simulink subsystem "ScannerBank"  (R2025b)
settings: Solver=VariableStepAuto  StartTime=0.0  StopTime=10.0  RelTol=1e-3
values from neighbouring files (symbols this model uses):
  m = min(v)    [run_loader_scanner_model_multi_stress_v1_2_final_verified.m]    (also in run_slide_model_daily_scenarios_v2.m; run_slide_model_daily_scenarios_v2_scannerbank_v2.m)
  ScannerEnabled = logical(S(testIdx).enabled(:).')    [run_loader_scanner_model_multi_stress_v1_2_final_verified.m]    (also in run_slide_model_daily_scenarios_v2_scannerbank_v2.m = false(1,n_physical_scanners))
  Total_Scanner_Rack_Slots_Available = nActiveScanners * Scanner_RackQueueSize    [run_loader_scanner_model_multi_stress_v1_2_final_verified.m]    (also in run_slide_model_daily_scenarios_v2.m = n_active_scanners * Scanner_RackQueueSize; run_slide_model_daily_scenarios_v2_scannerbank_v2.m = nnz(ScannerEnabled) * Scanner_RackQueueSize)
settings Model: Creator=bayes  LastModifiedBy=bayes

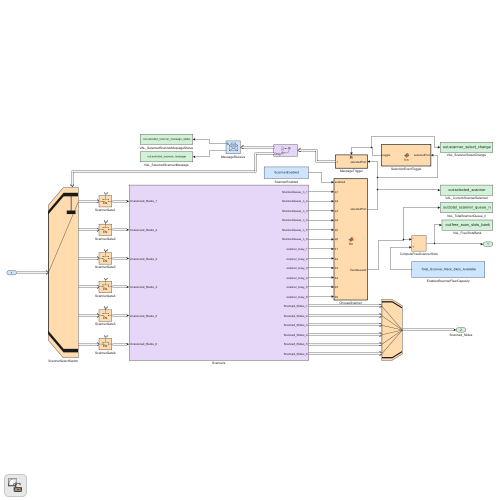
[thumbnail: Simulink's stored preview of the top-level diagram]
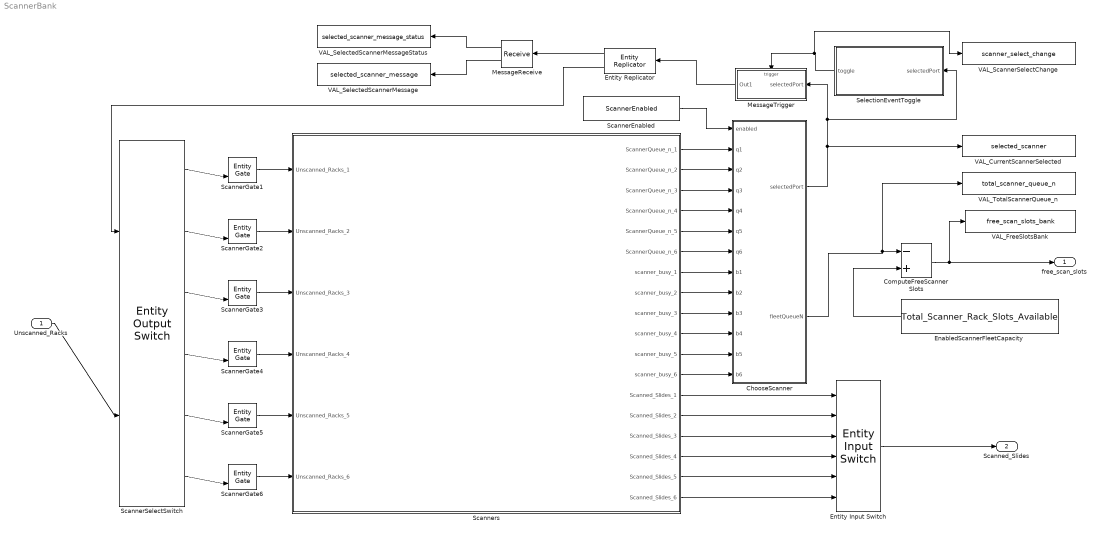
== system ScannerBank ==
  Unscanned_Racks : Inport
  ChooseScanner : MATLAB Function  TreatAsAtomicUnit=on
  ComputeFreeScannerSlots : Sum  Inputs=-+
  EnabledScannerFleetCapacity : Constant  Value=Total_Scanner_Rack_Slots_Available  OutMin=0
  Entity Input Switch : EntityInputSwitch  InputPortMessageModes=m,m,m,m,m,m  OutputPortMessageModes=m  NumberInputPorts=6
      settings: InputPortMap=u1,u2,u3,u4,u5,u6
  Entity Replicator : EntityReplicator  InputPortMessageModes=m  OutputPortMessageModes=m,m  HoldOriginalEntityUntilAllReplicasDepart=on
  MessageReceive : Receive  InputPortMessageModes=m  ShowQueueStatus=on  InitialValue=0  ValueSourceWhenQueueIsEmpty=Use initial value
      settings: OutputPortMap=o0,o1
  MessageTrigger : Subsystem  TreatAsAtomicUnit=on
  ScannerEnabled : Constant  Value=ScannerEnabled
  ScannerGate{1..6} (6 alike) : EntityGate  InputPortMessageModes=m,m  OutputPortMessageModes=m  OpenGateAtSimulationStart=on
  ScannerSelectSwitch : EntityOutputSwitch  InputPortMessageModes=m,m  OutputPortMessageModes=m,m,m,m,m,m  NumberOutputPorts=6  SwitchingCriterion=From control port  SwitchAttributeName=Attribute1
      settings: InputPortMap=u0,u1  OutputPortMap=o0,o1,o2,o3,o4,o5
  Scanners : Subsystem
  SelectionEventToggle : MATLAB Function  TreatAsAtomicUnit=on
  VAL_CurrentScannerSelected : ToWorkspace  VariableName=selected_scanner  SaveFormat=Timeseries  SampleTime=-1
  VAL_FreeSlotsBank : ToWorkspace  VariableName=free_scan_slots_bank  SaveFormat=Timeseries  SampleTime=-1
  VAL_ScannerSelectChange : ToWorkspace  VariableName=scanner_select_change  SaveFormat=Timeseries  SampleTime=-1
  VAL_SelectedScannerMessage : ToWorkspace  VariableName=selected_scanner_message  SaveFormat=Timeseries  SampleTime=-1
  VAL_SelectedScannerMessageStatus : ToWorkspace  VariableName=selected_scanner_message_status  SaveFormat=Timeseries  SampleTime=-1
  VAL_TotalScannerQueue_n : ToWorkspace  VariableName=total_scanner_queue_n  SaveFormat=Timeseries  SampleTime=-1
  free_scan_slots : Outport
  Scanned_Slides : Outport  Port=2
  wires:
  Scanners/2(ScannerQueue_n_2) -> ChooseScanner/3(q2)
  Scanners/9(scanner_busy_3) -> ChooseScanner/10(b3)
  Scanners/1(ScannerQueue_n_1) -> ChooseScanner/2(q1)
  Entity Replicator/2 -> ScannerSelectSwitch/1
  Scanners/16(Scanned_Slides_4) -> Entity Input Switch/4
  ScannerGate4/1 -> Scanners/4(Unscanned_Racks_4)
  Scanners/6(ScannerQueue_n_6) -> ChooseScanner/7(q6)
  MessageTrigger/1(Out1) -> Entity Replicator/1
  ScannerSelectSwitch/4 -> ScannerGate4/2
  ScannerSelectSwitch/6 -> ScannerGate6/2
  ScannerGate2/1 -> Scanners/2(Unscanned_Racks_2)
  ScannerGate1/1 -> Scanners/1(Unscanned_Racks_1)
  ChooseScanner/1(selectedPort) -> SelectionEventToggle/1(selectedPort), MessageTrigger/1(selectedPort), VAL_CurrentScannerSelected/1
  ScannerGate5/1 -> Scanners/5(Unscanned_Racks_5)
  Scanners/13(Scanned_Slides_1) -> Entity Input Switch/1
  EnabledScannerFleetCapacity/1 -> ComputeFreeScannerSlots/2
  ScannerSelectSwitch/5 -> ScannerGate5/2
  ScannerSelectSwitch/2 -> ScannerGate2/2
  Scanners/18(Scanned_Slides_6) -> Entity Input Switch/6
  Entity Input Switch/1 -> Scanned_Slides/1
  MessageReceive/1 -> VAL_SelectedScannerMessageStatus/1
  Entity Replicator/1 -> MessageReceive/1
  ScannerSelectSwitch/3 -> ScannerGate3/2
  Unscanned_Racks/1 -> ScannerSelectSwitch/2
  Scanners/5(ScannerQueue_n_5) -> ChooseScanner/6(q5)
  Scanners/11(scanner_busy_5) -> ChooseScanner/12(b5)
  ComputeFreeScannerSlots/1 -> free_scan_slots/1, VAL_FreeSlotsBank/1
  Scanners/14(Scanned_Slides_2) -> Entity Input Switch/2
  Scanners/8(scanner_busy_2) -> ChooseScanner/9(b2)
  ScannerSelectSwitch/1 -> ScannerGate1/2
  Scanners/12(scanner_busy_6) -> ChooseScanner/13(b6)
  MessageReceive/2 -> VAL_SelectedScannerMessage/1
  Scanners/4(ScannerQueue_n_4) -> ChooseScanner/5(q4)
  ScannerGate3/1 -> Scanners/3(Unscanned_Racks_3)
  Scanners/15(Scanned_Slides_3) -> Entity Input Switch/3
  Scanners/7(scanner_busy_1) -> ChooseScanner/8(b1)
  ChooseScanner/2(fleetQueueN) -> ComputeFreeScannerSlots/1, VAL_TotalScannerQueue_n/1
  Scanners/10(scanner_busy_4) -> ChooseScanner/11(b4)
  Scanners/17(Scanned_Slides_5) -> Entity Input Switch/5
  ScannerGate6/1 -> Scanners/6(Unscanned_Racks_6)
  ScannerEnabled/1 -> ChooseScanner/1(enabled)
  SelectionEventToggle/1(toggle) -> MessageTrigger/Trigger, VAL_ScannerSelectChange/1
  Scanners/3(ScannerQueue_n_3) -> ChooseScanner/4(q3)

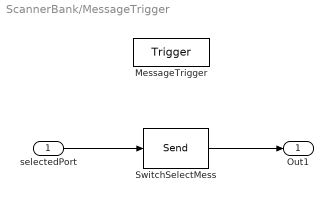
== system ScannerBank/MessageTrigger ==
  selectedPort : Inport
  MessageTrigger : TriggerPort  TriggerType=either  VariantControl=(inherit)
  SwitchSelectMess : Send  OutputPortMessageModes=m
  Out1 : Outport
  wires:
  SwitchSelectMess/1 -> Out1/1
  selectedPort/1 -> SwitchSelectMess/1

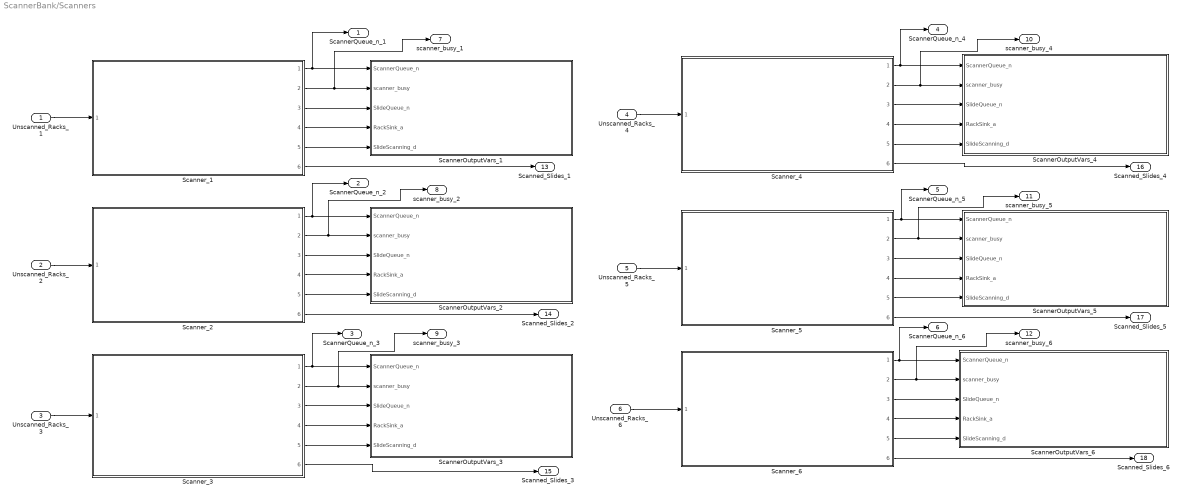
== system ScannerBank/Scanners ==
  Unscanned_Racks_1 : Inport
  Unscanned_Racks_2 : Inport  Port=2
  Unscanned_Racks_3 : Inport  Port=3
  Unscanned_Racks_4 : Inport  Port=4
  Unscanned_Racks_5 : Inport  Port=5
  Unscanned_Racks_6 : Inport  Port=6
  ScannerOutputVars_1 : Subsystem
  ScannerOutputVars_2 : Subsystem
  ScannerOutputVars_3 : Subsystem
  ScannerOutputVars_4 : Subsystem
  ScannerOutputVars_5 : Subsystem
  ScannerOutputVars_6 : Subsystem
  Scanner_{1..6} (6 alike) : Subsystem  ReferencedSubsystem=GenericScanner
  ScannerQueue_n_1 : Outport
  ScannerQueue_n_2 : Outport  Port=2
  ScannerQueue_n_3 : Outport  Port=3
  ScannerQueue_n_4 : Outport  Port=4
  ScannerQueue_n_5 : Outport  Port=5
  ScannerQueue_n_6 : Outport  Port=6
  scanner_busy_1 : Outport  Port=7
  scanner_busy_2 : Outport  Port=8
  scanner_busy_3 : Outport  Port=9
  scanner_busy_4 : Outport  Port=10
  scanner_busy_5 : Outport  Port=11
  scanner_busy_6 : Outport  Port=12
  Scanned_Slides_1 : Outport  Port=13
  Scanned_Slides_2 : Outport  Port=14
  Scanned_Slides_3 : Outport  Port=15
  Scanned_Slides_4 : Outport  Port=16
  Scanned_Slides_5 : Outport  Port=17
  Scanned_Slides_6 : Outport  Port=18
  wires:
  Scanner_2/6 -> Scanned_Slides_2/1
  Unscanned_Racks_4/1 -> Scanner_4/1
  Unscanned_Racks_1/1 -> Scanner_1/1
  Unscanned_Racks_6/1 -> Scanner_6/1
  Scanner_5/3 -> ScannerOutputVars_5/3(SlideQueue_n)
  Unscanned_Racks_3/1 -> Scanner_3/1
  Scanner_5/4 -> ScannerOutputVars_5/4(RackSink_a)
  Scanner_5/2 -> scanner_busy_5/1, ScannerOutputVars_5/2(scanner_busy)
  Scanner_2/4 -> ScannerOutputVars_2/4(RackSink_a)
  Scanner_1/6 -> Scanned_Slides_1/1
  Scanner_3/5 -> ScannerOutputVars_3/5(SlideScanning_d)
  Scanner_6/6 -> Scanned_Slides_6/1
  Scanner_3/4 -> ScannerOutputVars_3/4(RackSink_a)
  Scanner_1/3 -> ScannerOutputVars_1/3(SlideQueue_n)
  Scanner_6/4 -> ScannerOutputVars_6/4(RackSink_a)
  Scanner_2/2 -> scanner_busy_2/1, ScannerOutputVars_2/2(scanner_busy)
  Scanner_6/1 -> ScannerOutputVars_6/1(ScannerQueue_n), ScannerQueue_n_6/1
  Scanner_6/3 -> ScannerOutputVars_6/3(SlideQueue_n)
  Scanner_2/1 -> ScannerOutputVars_2/1(ScannerQueue_n), ScannerQueue_n_2/1
  Scanner_5/5 -> ScannerOutputVars_5/5(SlideScanning_d)
  Scanner_4/3 -> ScannerOutputVars_4/3(SlideQueue_n)
  Scanner_1/1 -> ScannerQueue_n_1/1, ScannerOutputVars_1/1(ScannerQueue_n)
  Scanner_6/5 -> ScannerOutputVars_6/5(SlideScanning_d)
  Scanner_4/1 -> ScannerOutputVars_4/1(ScannerQueue_n), ScannerQueue_n_4/1
  Scanner_4/5 -> ScannerOutputVars_4/5(SlideScanning_d)
  Scanner_3/2 -> ScannerOutputVars_3/2(scanner_busy), scanner_busy_3/1
  Unscanned_Racks_5/1 -> Scanner_5/1
  Scanner_6/2 -> scanner_busy_6/1, ScannerOutputVars_6/2(scanner_busy)
  Scanner_4/4 -> ScannerOutputVars_4/4(RackSink_a)
  Scanner_5/6 -> Scanned_Slides_5/1
  Scanner_3/6 -> Scanned_Slides_3/1
  Scanner_4/6 -> Scanned_Slides_4/1
  Scanner_1/2 -> ScannerOutputVars_1/2(scanner_busy), scanner_busy_1/1
  Scanner_5/1 -> ScannerOutputVars_5/1(ScannerQueue_n), ScannerQueue_n_5/1
  Scanner_4/2 -> scanner_busy_4/1, ScannerOutputVars_4/2(scanner_busy)
  Unscanned_Racks_2/1 -> Scanner_2/1
  Scanner_2/5 -> ScannerOutputVars_2/5(SlideScanning_d)
  Scanner_2/3 -> ScannerOutputVars_2/3(SlideQueue_n)
  Scanner_3/3 -> ScannerOutputVars_3/3(SlideQueue_n)
  Scanner_3/1 -> ScannerOutputVars_3/1(ScannerQueue_n), ScannerQueue_n_3/1
  Scanner_1/5 -> ScannerOutputVars_1/5(SlideScanning_d)
  Scanner_1/4 -> ScannerOutputVars_1/4(RackSink_a)

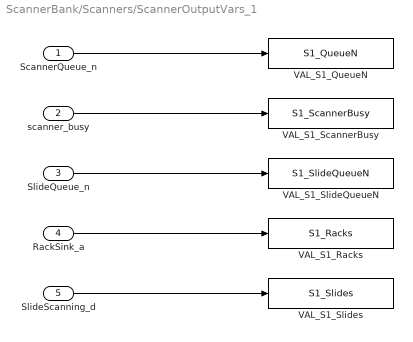
== system ScannerBank/Scanners/ScannerOutputVars_1 ==
  ScannerQueue_n : Inport
  scanner_busy : Inport  Port=2
  SlideQueue_n : Inport  Port=3
  RackSink_a : Inport  Port=4
  SlideScanning_d : Inport  Port=5
  VAL_S1_QueueN : ToWorkspace  VariableName=S1_QueueN  SaveFormat=Timeseries  SampleTime=-1
  VAL_S1_Racks : ToWorkspace  VariableName=S1_Racks  SaveFormat=Timeseries  SampleTime=-1
  VAL_S1_ScannerBusy : ToWorkspace  VariableName=S1_ScannerBusy  SaveFormat=Timeseries  SampleTime=-1
  VAL_S1_SlideQueueN : ToWorkspace  VariableName=S1_SlideQueueN  SaveFormat=Timeseries  SampleTime=-1
  VAL_S1_Slides : ToWorkspace  VariableName=S1_Slides  SaveFormat=Timeseries  SampleTime=-1
  wires:
  SlideScanning_d/1 -> VAL_S1_Slides/1
  SlideQueue_n/1 -> VAL_S1_SlideQueueN/1
  RackSink_a/1 -> VAL_S1_Racks/1
  ScannerQueue_n/1 -> VAL_S1_QueueN/1
  scanner_busy/1 -> VAL_S1_ScannerBusy/1

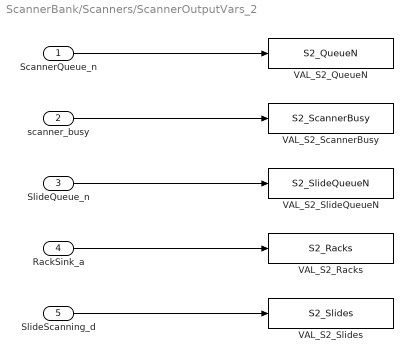
== system ScannerBank/Scanners/ScannerOutputVars_2 ==
  ScannerQueue_n : Inport
  scanner_busy : Inport  Port=2
  SlideQueue_n : Inport  Port=3
  RackSink_a : Inport  Port=4
  SlideScanning_d : Inport  Port=5
  VAL_S2_QueueN : ToWorkspace  VariableName=S2_QueueN  SaveFormat=Timeseries  SampleTime=-1
  VAL_S2_Racks : ToWorkspace  VariableName=S2_Racks  SaveFormat=Timeseries  SampleTime=-1
  VAL_S2_ScannerBusy : ToWorkspace  VariableName=S2_ScannerBusy  SaveFormat=Timeseries  SampleTime=-1
  VAL_S2_SlideQueueN : ToWorkspace  VariableName=S2_SlideQueueN  SaveFormat=Timeseries  SampleTime=-1
  VAL_S2_Slides : ToWorkspace  VariableName=S2_Slides  SaveFormat=Timeseries  SampleTime=-1
  wires:
  ScannerQueue_n/1 -> VAL_S2_QueueN/1
  SlideQueue_n/1 -> VAL_S2_SlideQueueN/1
  RackSink_a/1 -> VAL_S2_Racks/1
  SlideScanning_d/1 -> VAL_S2_Slides/1
  scanner_busy/1 -> VAL_S2_ScannerBusy/1

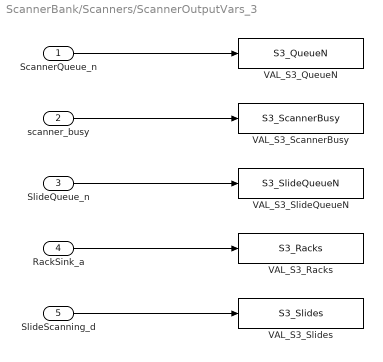
== system ScannerBank/Scanners/ScannerOutputVars_3 ==
  ScannerQueue_n : Inport
  scanner_busy : Inport  Port=2
  SlideQueue_n : Inport  Port=3
  RackSink_a : Inport  Port=4
  SlideScanning_d : Inport  Port=5
  VAL_S3_QueueN : ToWorkspace  VariableName=S3_QueueN  SaveFormat=Timeseries  SampleTime=-1
  VAL_S3_Racks : ToWorkspace  VariableName=S3_Racks  SaveFormat=Timeseries  SampleTime=-1
  VAL_S3_ScannerBusy : ToWorkspace  VariableName=S3_ScannerBusy  SaveFormat=Timeseries  SampleTime=-1
  VAL_S3_SlideQueueN : ToWorkspace  VariableName=S3_SlideQueueN  SaveFormat=Timeseries  SampleTime=-1
  VAL_S3_Slides : ToWorkspace  VariableName=S3_Slides  SaveFormat=Timeseries  SampleTime=-1
  wires:
  SlideScanning_d/1 -> VAL_S3_Slides/1
  RackSink_a/1 -> VAL_S3_Racks/1
  ScannerQueue_n/1 -> VAL_S3_QueueN/1
  SlideQueue_n/1 -> VAL_S3_SlideQueueN/1
  scanner_busy/1 -> VAL_S3_ScannerBusy/1

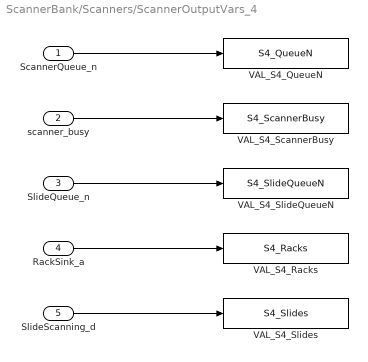
== system ScannerBank/Scanners/ScannerOutputVars_4 ==
  ScannerQueue_n : Inport
  scanner_busy : Inport  Port=2
  SlideQueue_n : Inport  Port=3
  RackSink_a : Inport  Port=4
  SlideScanning_d : Inport  Port=5
  VAL_S4_QueueN : ToWorkspace  VariableName=S4_QueueN  SaveFormat=Timeseries  SampleTime=-1
  VAL_S4_Racks : ToWorkspace  VariableName=S4_Racks  SaveFormat=Timeseries  SampleTime=-1
  VAL_S4_ScannerBusy : ToWorkspace  VariableName=S4_ScannerBusy  SaveFormat=Timeseries  SampleTime=-1
  VAL_S4_SlideQueueN : ToWorkspace  VariableName=S4_SlideQueueN  SaveFormat=Timeseries  SampleTime=-1
  VAL_S4_Slides : ToWorkspace  VariableName=S4_Slides  SaveFormat=Timeseries  SampleTime=-1
  wires:
  ScannerQueue_n/1 -> VAL_S4_QueueN/1
  SlideQueue_n/1 -> VAL_S4_SlideQueueN/1
  SlideScanning_d/1 -> VAL_S4_Slides/1
  RackSink_a/1 -> VAL_S4_Racks/1
  scanner_busy/1 -> VAL_S4_ScannerBusy/1

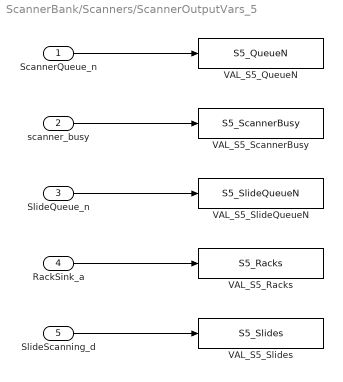
== system ScannerBank/Scanners/ScannerOutputVars_5 ==
  ScannerQueue_n : Inport
  scanner_busy : Inport  Port=2
  SlideQueue_n : Inport  Port=3
  RackSink_a : Inport  Port=4
  SlideScanning_d : Inport  Port=5
  VAL_S5_QueueN : ToWorkspace  VariableName=S5_QueueN  SaveFormat=Timeseries  SampleTime=-1
  VAL_S5_Racks : ToWorkspace  VariableName=S5_Racks  SaveFormat=Timeseries  SampleTime=-1
  VAL_S5_ScannerBusy : ToWorkspace  VariableName=S5_ScannerBusy  SaveFormat=Timeseries  SampleTime=-1
  VAL_S5_SlideQueueN : ToWorkspace  VariableName=S5_SlideQueueN  SaveFormat=Timeseries  SampleTime=-1
  VAL_S5_Slides : ToWorkspace  VariableName=S5_Slides  SaveFormat=Timeseries  SampleTime=-1
  wires:
  ScannerQueue_n/1 -> VAL_S5_QueueN/1
  SlideQueue_n/1 -> VAL_S5_SlideQueueN/1
  RackSink_a/1 -> VAL_S5_Racks/1
  SlideScanning_d/1 -> VAL_S5_Slides/1
  scanner_busy/1 -> VAL_S5_ScannerBusy/1

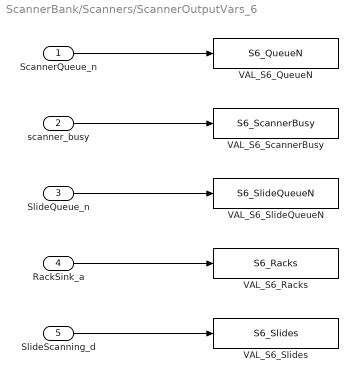
== system ScannerBank/Scanners/ScannerOutputVars_6 ==
  ScannerQueue_n : Inport
  scanner_busy : Inport  Port=2
  SlideQueue_n : Inport  Port=3
  RackSink_a : Inport  Port=4
  SlideScanning_d : Inport  Port=5
  VAL_S6_QueueN : ToWorkspace  VariableName=S6_QueueN  SaveFormat=Timeseries  SampleTime=-1
  VAL_S6_Racks : ToWorkspace  VariableName=S6_Racks  SaveFormat=Timeseries  SampleTime=-1
  VAL_S6_ScannerBusy : ToWorkspace  VariableName=S6_ScannerBusy  SaveFormat=Timeseries  SampleTime=-1
  VAL_S6_SlideQueueN : ToWorkspace  VariableName=S6_SlideQueueN  SaveFormat=Timeseries  SampleTime=-1
  VAL_S6_Slides : ToWorkspace  VariableName=S6_Slides  SaveFormat=Timeseries  SampleTime=-1
  wires:
  ScannerQueue_n/1 -> VAL_S6_QueueN/1
  SlideQueue_n/1 -> VAL_S6_SlideQueueN/1
  SlideScanning_d/1 -> VAL_S6_Slides/1
  RackSink_a/1 -> VAL_S6_Racks/1
  scanner_busy/1 -> VAL_S6_ScannerBusy/1

== matlab function ScannerBank/SelectionEventToggle ==
  data: selectedPort input; toggle output
function toggle = fcn(selectedPort)
%#codegen

persistent lastPort toggleState

if isempty(lastPort)
    lastPort    = uint8(1);
    toggleState = uint8(0);
end

if selectedPort ~= lastPort
    toggleState = uint8(1) - toggleState;
    lastPort = selectedPort;
end

toggle = toggleState;

== matlab function ScannerBank/ChooseScanner ==
  data: enabled input; q1 input; q2 input; selectedPort output; fleetQueueN output; q3 input; q4 input; q5 input; q6 input; b1 input; b2 input; b3 input; b4 input; b5 input; b6 input
function [selectedPort, fleetQueueN] = fcn( ...
    enabled, ...
    q1, q2, q3, q4, q5, q6, ...
    b1, b2, b3, b4, b5, b6)
%#codegen
%
% v1.2 scanner routing policy
%
% Inputs:
%   enabled = 6-element logical vector
%   q1-q6   = ScannerQueue_n for scanners 1-6
%   b1-b6   = scanner_busy for scanners 1-6
%
% Outputs:
%   selectedPort = scanner number, 1-6
%   fleetQueueN  = total ScannerQueue occupancy
%
% Routing:
%   1. Choose first enabled scanner that is not busy.
%   2. If all enabled scanners are busy, choose the enabled
%      scanner with the smallest ScannerQueue occupancy.
%   3. Ties go to the lowest-numbered scanner.
%
% v1.2 design rule:
%   Scanner 1 is always enabled.

%% Assemble local state vectors
queueN = [q1 q2 q3 q4 q5 q6];
busy   = [b1 b2 b3 b4 b5 b6];

%% Fleet queue occupancy
fleetQueueN = q1 + q2 + q3 + q4 + q5 + q6;

%% Safe initial/default selection
selectedPort = uint8(1);

%% Priority 1: first enabled scanner that is not busy
for i = 1:6
    if enabled(i) && ~busy(i)
        selectedPort = uint8(i);
        return;
    end
end

%% Priority 2: all enabled scanners are busy
% Choose enabled scanner with smallest rack queue.
bestQueue = inf;

for i = 1:6
    if enabled(i) && queueN(i) < bestQueue
        bestQueue = queueN(i);
        selectedPort = uint8(i);
    end
end

end
